simulink model "tankfnc"  (R2018b)
settings: Solver=ode1  StartTime=0.0  StopTime=100  RelTol=1e-3
values from neighbouring files (symbols this model uses):
  qzu = 5    [gastank.m]    (also in tank.m)
settings Model: Creator=Naveen  LastModifiedBy=Naveen

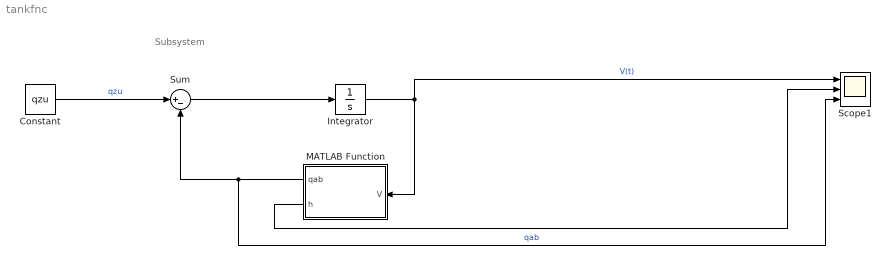
== system tankfnc ==
  note: Subsystem
  Constant : Constant  Value=qzu
  Integrator : Integrator
  MATLAB Function : MATLAB Function  TreatAsAtomicUnit=on
  Scope1 : Scope  NumInputPorts=3
  Sum : Sum  Inputs=|+-
  wires:
  MATLAB Function/1(qab) -> Sum/2, Scope1/3  "qab"
  Integrator/1 -> Scope1/1, MATLAB Function/1(V)  "V(t)"
  Constant/1 -> Sum/1  "qzu"
  Sum/1 -> Integrator/1
  MATLAB Function/2(h) -> Scope1/2

== matlab function tankfnc/MATLAB Function ==
  data: V input; qab output; h output
function [qab,h] = tankfnc(V)
A=3;
a=0.3;
g=9.81;
qzu=5;
h=V/A;
qab=a*(sqrt(2*g*h));
